simulink model "gm_motor_dtf_antiwindup_vnl"  (R2021b)
settings: Solver=FixedStepDiscrete  StartTime=0.0  StopTime=10  RelTol=1e-3
undefined symbols (not defined in the file or in its folder): DiscIntNeverNeededParam
libraries: simulink x5
Description:
  | Symmetric FIR Filter
  | This example shows how to use HDL Coder(TM) to check, generate,
  | and verify HDL for a fixed-point symmetric FIR filter.
settings Model: Creator=The MathWorks, Inc.  LastModifiedBy=Marco Milanesi
settings SolverCC: AlgebraicLoopSolver=TrustRegion  AutoInsertRateTranBlk=on
settings DataIOCC: LimitDataPoints=on  SaveFormat=Array  SaveOutput=off  SignalLogging=off  SaveTime=off  ReturnWorkspaceOutputs=off  SignalLoggingName=logsOut
settings OptimizationCC: BlockReduction=off  BooleanDataType=off  ConditionallyExecuteInputs=off  DefaultParameterBehavior=Inlined  InheritOutputTypeSmallerThanSingle=on  InlineInvariantSignals=on  ExpressionDepthLimit=2147483647  InitFltsAndDblsToZero=on  LifeSpan=inf  BufferReusableBoundary=off
settings DebuggingCC: AlgebraicLoopMsg=error  SaveWithParameterizedLinksMsg=none  UnderspecifiedInitializationDetection=Classic  MergeDetectMultiDrivingBlocksExec=none  CheckExecutionContextPreStartOutputMsg=on  SignalResolutionControl=TryResolveAllWithWarning  InheritedTsInSrcMsg=none  MultiTaskDSMMsg=warning  MultiTaskCondExecSysMsg=none  SingleTaskRateTransMsg=error  IntegerOverflowMsg=none  ParameterPrecisionLossMsg=none  FcnCallInpInsideContextMsg=warning  BusObjectLabelMismatch=none  StateNameClashWarn=warning  SFUnexpectedBacktrackingDiag=warning  SFNoUnconditionalDefaultTransitionDiag=warning  SFExecutionAtInitializationDiag=none  SFMachineParentedDataDiag=warning  IntegerSaturationMsg=none  ArithmeticOperatorsInVariantConditions=warning
settings HardwareCC: ProdBitPerPointer=32  ProdBitPerSizeT=32  ProdBitPerPtrDiffT=32  ProdLargestAtomicFloat=None  ProdIntDivRoundTo=Undefined  ProdEndianess=Unspecified  ProdWordSize=32  ProdHWDeviceType=ASIC/FPGA  TargetUnknown=on  ProdEqTarget=off
settings ModelReferenceCC: PropagateSignalLabelsOutOfModel=off
settings SFSimCC: SimUseLocalCustomCode=off  CustomCodeUndefinedFunction=UseInterfaceOnly
settings RTWCC: RTWUseLocalCustomCode=off
settings CodeAppCC: StateflowObjectComments=on
settings GRTTargetCC: TargetFcnLib=ansi_tfl_tmw.mat  TargetLangStandard=C89/C90 (ANSI)  CombineOutputUpdateFcns=off  GRTInterface=on
settings ConfigComp: CovMetricSettings=dw  CovSaveCumulativeToWorkspaceVar=on  CovSaveSingleToWorkspaceVar=on  CovExternalEMLEnable=off

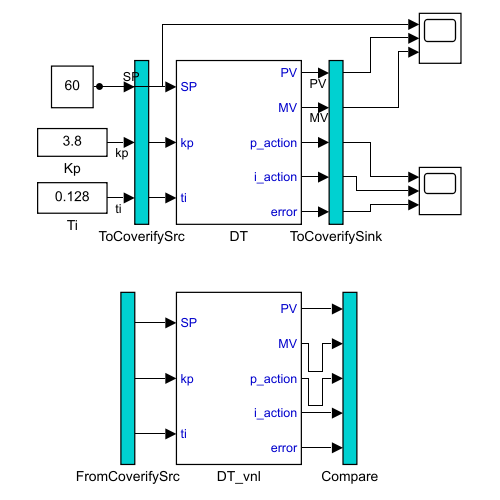
[thumbnail: Simulink's stored preview of the top-level diagram]
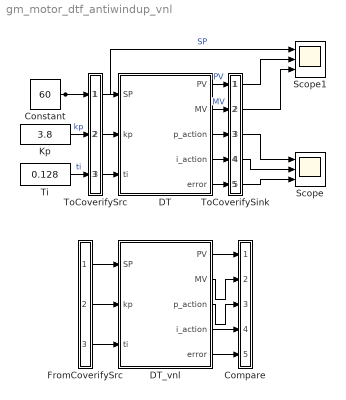
== system gm_motor_dtf_antiwindup_vnl ==
  Compare : Subsystem
      mask Display: disp('')
  Constant : Constant  Value=60  OutDataTypeStr=fixdt(1,10,0)
  DT : Subsystem
  DT_vnl : Subsystem
  FromCoverifySrc : Subsystem
      mask Display: disp('')
  Kp : Constant  Value=3.8  OutDataTypeStr=fixdt(1,10,0)
  Scope : Scope  NumInputPorts=3
  Scope1 : Scope  NumInputPorts=3
  Ti : Constant  Value=0.128  OutDataTypeStr=fixdt(1,10,0)
  ToCoverifySink : Subsystem
      mask Display: disp('')
  ToCoverifySrc : Subsystem
      mask Display: disp('')
  wires:
  Constant/1 -> Scope1/1, ToCoverifySrc/1(in1)  "SP"
  ToCoverifySrc/1(out1) -> DT/1(SP)
  ToCoverifySrc/2(out2) -> DT/2(kp)
  ToCoverifySrc/3(out3) -> DT/3(ti)
  DT/1(PV) -> ToCoverifySink/1(in1)  "PV"
  DT/2(MV) -> ToCoverifySink/2(in2)  "MV"
  DT/3(p_action) -> ToCoverifySink/3(in3)
  DT/4(i_action) -> ToCoverifySink/4(in4)
  DT/5(error) -> ToCoverifySink/5(in5)
  Kp/1 -> ToCoverifySrc/2(in2)  "kp"
  Ti/1 -> ToCoverifySrc/3(in3)  "ti"
  ToCoverifySink/1(out1) -> Scope1/2
  ToCoverifySink/2(out2) -> Scope1/3
  ToCoverifySink/3(out3) -> Scope/1
  ToCoverifySink/4(out4) -> Scope/2
  ToCoverifySink/5(out5) -> Scope/3
  FromCoverifySrc/1(out1) -> DT_vnl/1(SP)
  FromCoverifySrc/2(out2) -> DT_vnl/2(kp)
  FromCoverifySrc/3(out3) -> DT_vnl/3(ti)
  DT_vnl/1(PV) -> Compare/1(in1)
  DT_vnl/2(MV) -> Compare/2(in2)
  DT_vnl/3(p_action) -> Compare/3(in3)
  DT_vnl/4(i_action) -> Compare/4(in4)
  DT_vnl/5(error) -> Compare/5(in5)

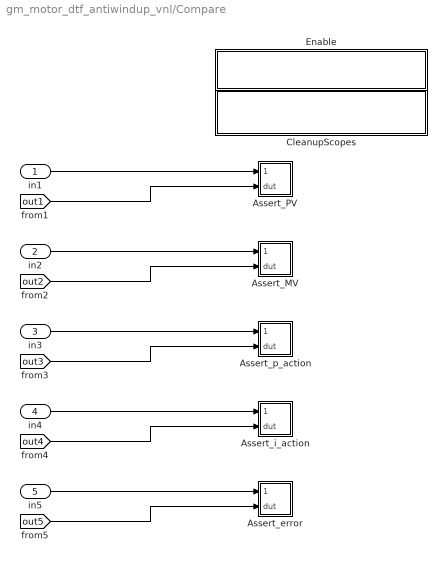
== system gm_motor_dtf_antiwindup_vnl/Compare ==
  in1 : Inport
  in2 : Inport  Port=2
  in3 : Inport  Port=3
  in4 : Inport  Port=4
  in5 : Inport  Port=5
  Assert_MV : Subsystem
  Assert_PV : Subsystem
  Assert_error : Subsystem
  Assert_i_action : Subsystem
  Assert_p_action : Subsystem
  CleanupScopes : Subsystem
      settings: OpenFcn=|
      | blkName = gcb; %self block
      | idx = regexp(blkName, '/CleanupScopes$', 'once');
      | blkParent = blkName(1:idx-1);
      | blks=find_system(blkParent, 'LookUnderMasks', 'all','blocktype', 'Scope');
      | for itr = 1:length(blks)
      | 	 hScopeCfg = get_param(blks{itr},'ScopeConfiguration');
      | 	 hScopeCfg.Visible = ~ hScopeCfg.Visible;
      | end
      | drawnow;
      mask Display: fprintf(message('hdlcoder:cosim:vnl_dblclick').getString());
  Enable : Subsystem
      settings: OpenFcn=|
      | blkName = gcb;
      | idx = regexp(blkName, '/Enable$', 'once');
      | blkParent = blkName(1:idx-1);
      | blks=find_system(blkParent, 'LookUnderMasks', 'all','blocktype', 'Assertion');
      | e = get_param(blks{1}, 'Enabled');
      | if strcmp(e, 'on'), f= 'off';, else, f = 'on';, end
      | for ii=1:length(blks), set_param(blks{ii}, 'Enabled', f);, end
      | set_param(gcb, 'MaskDisplay',['fprintf(message(''hdlcoder:cosim:vnl_dblclick_assertions'',','''',upper(e),'''',').getString())']);
      mask Display: fprintf(message('hdlcoder:cosim:vnl_dblclick_assertions','OFF').getString());
  wires:
  in1/1 -> Assert_PV/1(cosim)
  [out1] -> Assert_PV/2(dut)
  in2/1 -> Assert_MV/1(cosim)
  [out2] -> Assert_MV/2(dut)
  in3/1 -> Assert_p_action/1(cosim)
  [out3] -> Assert_p_action/2(dut)
  in4/1 -> Assert_i_action/1(cosim)
  [out4] -> Assert_i_action/2(dut)
  in5/1 -> Assert_error/1(cosim)
  [out5] -> Assert_error/2(dut)

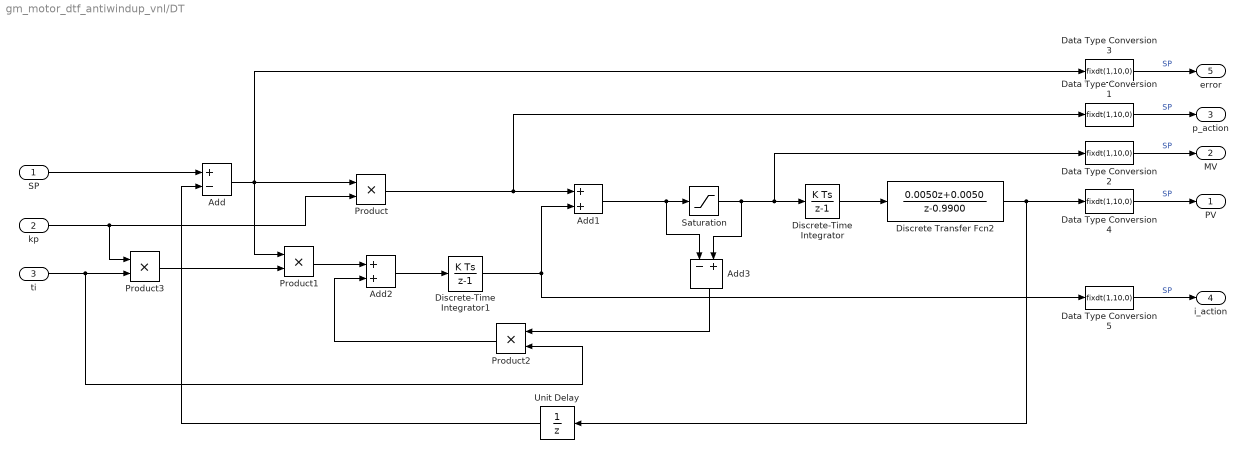
== system gm_motor_dtf_antiwindup_vnl/DT ==
  SP : Inport
  kp : Inport  Port=2
  ti : Inport  Port=3
  Add : Sum  Inputs=+-  AccumDataTypeStr=fixdt(1,64,32)  OutDataTypeStr=fixdt(1,64,32)
  Add1 : Sum  AccumDataTypeStr=fixdt(1,64,32)  OutDataTypeStr=fixdt(1,64,32)
  Add2 : Sum  AccumDataTypeStr=fixdt(1,64,32)  OutDataTypeStr=fixdt(1,64,32)
  Add3 : Sum  Inputs=-+  AccumDataTypeStr=fixdt(1,64,32)  OutDataTypeStr=fixdt(1,64,32)
  Data Type Conversion{1..5} (5 alike) : DataTypeConversion  OutDataTypeStr=fixdt(1,10,0)
  Discrete Transfer Fcn2 : DiscreteTransferFcn  Numerator=[0.0050 0.0050]  Denominator=[1 -0.9900]  SampleTime=0.0001  NumCoefDataTypeStr=fixdt(1,64,32)  DenCoefDataTypeStr=fixdt(1,64,32)  NumProductDataTypeStr=fixdt(1,64,32)  DenProductDataTypeStr=fixdt(1,64,32)  NumAccumDataTypeStr=fixdt(1,64,32)  DenAccumDataTypeStr=fixdt(1,64,32)  OutDataTypeStr=fixdt(1,64,32)
  Discrete-Time Integrator : DiscreteIntegrator  SampleTime=0.0001  OutDataTypeStr=fixdt(1,64,32)  ICPrevOutput=DiscIntNeverNeededParam  ICPrevScaledInput=DiscIntNeverNeededParam
  Discrete-Time Integrator1 : DiscreteIntegrator  SampleTime=0.0001  OutDataTypeStr=fixdt(1,64,32)  ICPrevOutput=DiscIntNeverNeededParam  ICPrevScaledInput=DiscIntNeverNeededParam
  Product : Product  OutDataTypeStr=fixdt(1,64,32)
  Product1 : Product  OutDataTypeStr=fixdt(1,64,32)
  Product2 : Product  OutDataTypeStr=fixdt(1,64,32)
  Product3 : Product
  Saturation : Saturate  UpperLimit=255  LowerLimit=-255  OutDataTypeStr=fixdt(1,64,32)
  Unit Delay : UnitDelay  SampleTime=0.0001  HasFrameUpgradeWarning=on
  PV : Outport  OutDataTypeStr=fixdt(1,10,0)  SampleTime=0.001  VectorParamsAs1DForOutWhenUnconnected=off
  MV : Outport  Port=2  OutDataTypeStr=fixdt(1,10,0)  SampleTime=0.001  VectorParamsAs1DForOutWhenUnconnected=off
  p_action : Outport  Port=3  OutDataTypeStr=fixdt(1,10,0)  SampleTime=0.001  VectorParamsAs1DForOutWhenUnconnected=off
  i_action : Outport  Port=4  OutDataTypeStr=fixdt(1,10,0)  SampleTime=0.001  VectorParamsAs1DForOutWhenUnconnected=off
  error : Outport  Port=5  OutDataTypeStr=fixdt(1,10,0)  SampleTime=0.001  VectorParamsAs1DForOutWhenUnconnected=off
  wires:
  SP/1 -> Add/1
  Discrete Transfer Fcn2/1 -> Data Type Conversion4/1, Unit Delay/1
  Add/1 -> Data Type Conversion3/1, Product/1, Product1/1
  kp/1 -> Product3/1, Product/2
  Product/1 -> Data Type Conversion1/1, Add1/1
  Discrete-Time Integrator1/1 -> Data Type Conversion5/1, Add1/2
  Discrete-Time Integrator/1 -> Discrete Transfer Fcn2/1
  Unit Delay/1 -> Add/2
  Saturation/1 -> Data Type Conversion2/1, Discrete-Time Integrator/1, Add3/2
  Add1/1 -> Add3/1, Saturation/1
  Product1/1 -> Add2/1
  Add2/1 -> Discrete-Time Integrator1/1
  Add3/1 -> Product2/1
  Product2/1 -> Add2/2
  ti/1 -> Product3/2, Product2/2
  Product3/1 -> Product1/2
  Data Type Conversion3/1 -> error/1  "SP"
  Data Type Conversion1/1 -> p_action/1  "SP"
  Data Type Conversion4/1 -> PV/1  "SP"
  Data Type Conversion2/1 -> MV/1  "SP"
  Data Type Conversion5/1 -> i_action/1  "SP"

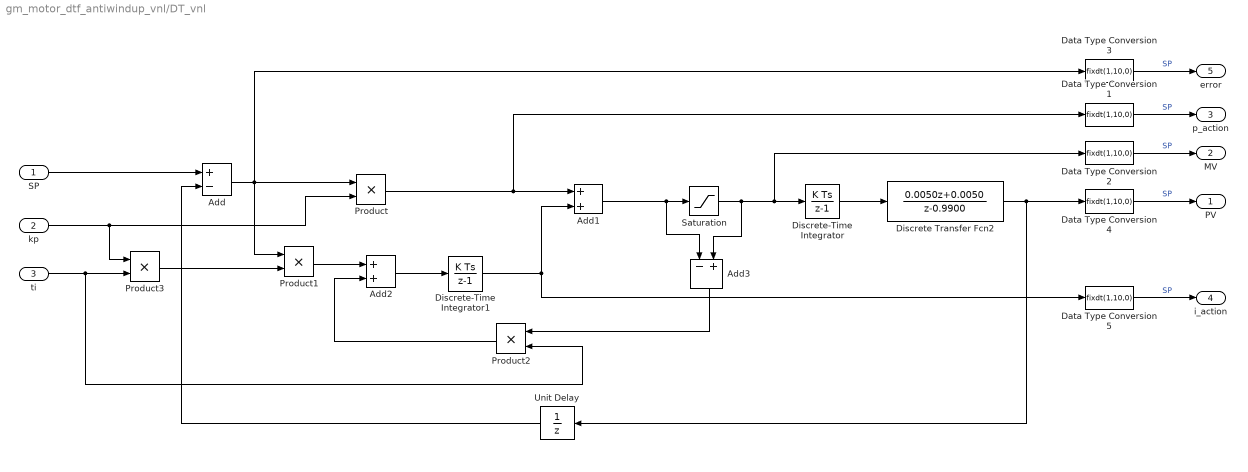
== system gm_motor_dtf_antiwindup_vnl/DT_vnl ==
  SP : Inport
  kp : Inport  Port=2
  ti : Inport  Port=3
  Add : Sum  Inputs=+-  AccumDataTypeStr=fixdt(1,64,32)  OutDataTypeStr=fixdt(1,64,32)
  Add1 : Sum  AccumDataTypeStr=fixdt(1,64,32)  OutDataTypeStr=fixdt(1,64,32)
  Add2 : Sum  AccumDataTypeStr=fixdt(1,64,32)  OutDataTypeStr=fixdt(1,64,32)
  Add3 : Sum  Inputs=-+  AccumDataTypeStr=fixdt(1,64,32)  OutDataTypeStr=fixdt(1,64,32)
  Data Type Conversion{1..5} (5 alike) : DataTypeConversion  OutDataTypeStr=fixdt(1,10,0)
  Discrete Transfer Fcn2 : DiscreteTransferFcn  Numerator=[0.0050 0.0050]  Denominator=[1 -0.9900]  SampleTime=0.0001  NumCoefDataTypeStr=fixdt(1,64,32)  DenCoefDataTypeStr=fixdt(1,64,32)  NumProductDataTypeStr=fixdt(1,64,32)  DenProductDataTypeStr=fixdt(1,64,32)  NumAccumDataTypeStr=fixdt(1,64,32)  DenAccumDataTypeStr=fixdt(1,64,32)  OutDataTypeStr=fixdt(1,64,32)
  Discrete-Time Integrator : DiscreteIntegrator  SampleTime=0.0001  OutDataTypeStr=fixdt(1,64,32)  ICPrevOutput=DiscIntNeverNeededParam  ICPrevScaledInput=DiscIntNeverNeededParam
  Discrete-Time Integrator1 : DiscreteIntegrator  SampleTime=0.0001  OutDataTypeStr=fixdt(1,64,32)  ICPrevOutput=DiscIntNeverNeededParam  ICPrevScaledInput=DiscIntNeverNeededParam
  Product : Product  OutDataTypeStr=fixdt(1,64,32)
  Product1 : Product  OutDataTypeStr=fixdt(1,64,32)
  Product2 : Product  OutDataTypeStr=fixdt(1,64,32)
  Product3 : Product
  Saturation : Saturate  UpperLimit=255  LowerLimit=-255  OutDataTypeStr=fixdt(1,64,32)
  Unit Delay : UnitDelay  SampleTime=0.0001  HasFrameUpgradeWarning=on
  PV : Outport  OutDataTypeStr=fixdt(1,10,0)  SampleTime=0.001  VectorParamsAs1DForOutWhenUnconnected=off
  MV : Outport  Port=2  OutDataTypeStr=fixdt(1,10,0)  SampleTime=0.001  VectorParamsAs1DForOutWhenUnconnected=off
  p_action : Outport  Port=3  OutDataTypeStr=fixdt(1,10,0)  SampleTime=0.001  VectorParamsAs1DForOutWhenUnconnected=off
  i_action : Outport  Port=4  OutDataTypeStr=fixdt(1,10,0)  SampleTime=0.001  VectorParamsAs1DForOutWhenUnconnected=off
  error : Outport  Port=5  OutDataTypeStr=fixdt(1,10,0)  SampleTime=0.001  VectorParamsAs1DForOutWhenUnconnected=off
  wires:
  Data Type Conversion5/1 -> i_action/1  "SP"
  Data Type Conversion2/1 -> MV/1  "SP"
  Data Type Conversion4/1 -> PV/1  "SP"
  Data Type Conversion1/1 -> p_action/1  "SP"
  Data Type Conversion3/1 -> error/1  "SP"
  Product3/1 -> Product1/2
  ti/1 -> Product2/2, Product3/2
  Product2/1 -> Add2/2
  Add3/1 -> Product2/1
  Add2/1 -> Discrete-Time Integrator1/1
  Product1/1 -> Add2/1
  Add1/1 -> Saturation/1, Add3/1
  Saturation/1 -> Add3/2, Discrete-Time Integrator/1, Data Type Conversion2/1
  Unit Delay/1 -> Add/2
  Discrete-Time Integrator/1 -> Discrete Transfer Fcn2/1
  Discrete-Time Integrator1/1 -> Add1/2, Data Type Conversion5/1
  Product/1 -> Add1/1, Data Type Conversion1/1
  kp/1 -> Product/2, Product3/1
  Add/1 -> Product1/1, Product/1, Data Type Conversion3/1
  Discrete Transfer Fcn2/1 -> Unit Delay/1, Data Type Conversion4/1
  SP/1 -> Add/1

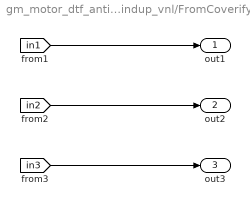
== system gm_motor_dtf_antiwindup_vnl/FromCoverifySrc ==
  out1 : Outport
  out2 : Outport  Port=2
  out3 : Outport  Port=3
  wires:
  [in1] -> out1/1
  [in2] -> out2/1
  [in3] -> out3/1

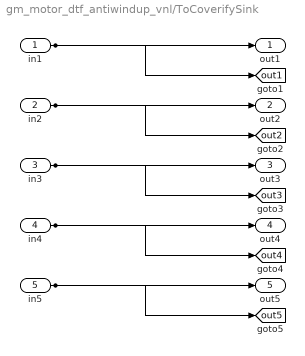
== system gm_motor_dtf_antiwindup_vnl/ToCoverifySink ==
  in1 : Inport
  in2 : Inport  Port=2
  in3 : Inport  Port=3
  in4 : Inport  Port=4
  in5 : Inport  Port=5
  out1 : Outport
  out2 : Outport  Port=2
  out3 : Outport  Port=3
  out4 : Outport  Port=4
  out5 : Outport  Port=5
  tag scope: out1=global, out2=global, out3=global, out4=global, out5=global
  wires:
  in1/1 -> out1/1, [out1]
  in2/1 -> out2/1, [out2]
  in3/1 -> out3/1, [out3]
  in4/1 -> out4/1, [out4]
  in5/1 -> out5/1, [out5]

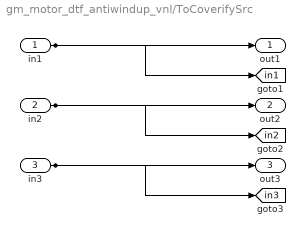
== system gm_motor_dtf_antiwindup_vnl/ToCoverifySrc ==
  in1 : Inport
  in2 : Inport  Port=2
  in3 : Inport  Port=3
  out1 : Outport
  out2 : Outport  Port=2
  out3 : Outport  Port=3
  tag scope: in1=global, in2=global, in3=global
  wires:
  in1/1 -> out1/1, [in1]
  in2/1 -> out2/1, [in2]
  in3/1 -> out3/1, [in3]

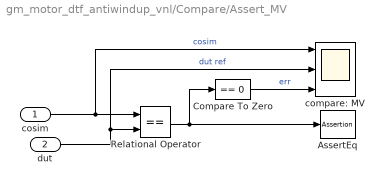
== system gm_motor_dtf_antiwindup_vnl/Compare/Assert_MV ==
  cosim : Inport
  dut : Inport  Port=2
  AssertEq : Assertion  StopWhenAssertionFail=off
  Compare To Zero : simulink/Logic and Bit Operations/Compare To Zero  relop===  OutDataTypeStr=boolean
  Relational Operator : RelationalOperator  Operator===  OutDataTypeStr=boolean  RndMeth=Nearest
  compare: MV : Scope  NumInputPorts=3
  wires:
  Compare To Zero/1 -> compare: MV/3  "err"
  Relational Operator/1 -> Compare To Zero/1, AssertEq/1
  cosim/1 -> compare: MV/1, Relational Operator/1  "cosim"
  dut/1 -> compare: MV/2, Relational Operator/2  "dut ref"

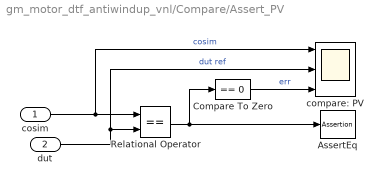
== system gm_motor_dtf_antiwindup_vnl/Compare/Assert_PV ==
  cosim : Inport
  dut : Inport  Port=2
  AssertEq : Assertion  StopWhenAssertionFail=off
  Compare To Zero : simulink/Logic and Bit Operations/Compare To Zero  relop===  OutDataTypeStr=boolean
  Relational Operator : RelationalOperator  Operator===  OutDataTypeStr=boolean  RndMeth=Nearest
  compare: PV : Scope  NumInputPorts=3
  wires:
  Compare To Zero/1 -> compare: PV/3  "err"
  Relational Operator/1 -> Compare To Zero/1, AssertEq/1
  cosim/1 -> compare: PV/1, Relational Operator/1  "cosim"
  dut/1 -> compare: PV/2, Relational Operator/2  "dut ref"

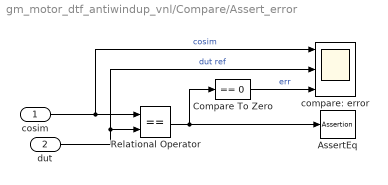
== system gm_motor_dtf_antiwindup_vnl/Compare/Assert_error ==
  cosim : Inport
  dut : Inport  Port=2
  AssertEq : Assertion  StopWhenAssertionFail=off
  Compare To Zero : simulink/Logic and Bit Operations/Compare To Zero  relop===  OutDataTypeStr=boolean
  Relational Operator : RelationalOperator  Operator===  OutDataTypeStr=boolean  RndMeth=Nearest
  compare: error : Scope  NumInputPorts=3
  wires:
  Compare To Zero/1 -> compare: error/3  "err"
  Relational Operator/1 -> Compare To Zero/1, AssertEq/1
  cosim/1 -> compare: error/1, Relational Operator/1  "cosim"
  dut/1 -> compare: error/2, Relational Operator/2  "dut ref"

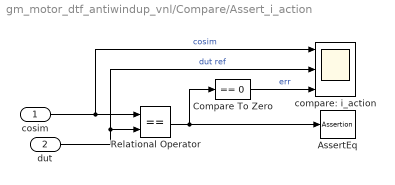
== system gm_motor_dtf_antiwindup_vnl/Compare/Assert_i_action ==
  cosim : Inport
  dut : Inport  Port=2
  AssertEq : Assertion  StopWhenAssertionFail=off
  Compare To Zero : simulink/Logic and Bit Operations/Compare To Zero  relop===  OutDataTypeStr=boolean
  Relational Operator : RelationalOperator  Operator===  OutDataTypeStr=boolean  RndMeth=Nearest
  compare: i_action : Scope  NumInputPorts=3
  wires:
  Compare To Zero/1 -> compare: i_action/3  "err"
  Relational Operator/1 -> Compare To Zero/1, AssertEq/1
  cosim/1 -> compare: i_action/1, Relational Operator/1  "cosim"
  dut/1 -> compare: i_action/2, Relational Operator/2  "dut ref"

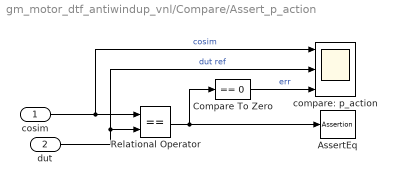
== system gm_motor_dtf_antiwindup_vnl/Compare/Assert_p_action ==
  cosim : Inport
  dut : Inport  Port=2
  AssertEq : Assertion  StopWhenAssertionFail=off
  Compare To Zero : simulink/Logic and Bit Operations/Compare To Zero  relop===  OutDataTypeStr=boolean
  Relational Operator : RelationalOperator  Operator===  OutDataTypeStr=boolean  RndMeth=Nearest
  compare: p_action : Scope  NumInputPorts=3
  wires:
  Compare To Zero/1 -> compare: p_action/3  "err"
  Relational Operator/1 -> Compare To Zero/1, AssertEq/1
  cosim/1 -> compare: p_action/1, Relational Operator/1  "cosim"
  dut/1 -> compare: p_action/2, Relational Operator/2  "dut ref"

== system gm_motor_dtf_antiwindup_vnl/Compare/CleanupScopes ==

== system gm_motor_dtf_antiwindup_vnl/Compare/Enable ==
